simulink model "SimulationDroneSetup"  (R2025a)
settings: Solver=ode15s  StartTime=0.0  StopTime=3  FixedStep=0.03  RelTol=1e-3
InitFcn:
  | %% System Constants
  | 
  | % mass
  | m = 0.12635;
  | 
  | % graviational constant
  | g = 9.81;
  | 
  | % Moment of inertia
  | I_XX = 0.00016159;
  | I_YY = 0.00016466;
  | I_ZZ = 0.00026144;
  | 
  | % thrust and power factor - needs to be measured
  | c_t = 2.07732E-05;
  | c_p = 2.76277E-06;
  | 
  | % https://en.wikipedia.org/wiki/Density_of_air
  | rho = 1.225;
  | 
  | % surface area of a propeller - estimation based on half of circle area
  | diameter = 0.04;
  | A = pi * (diameter/2)^2 / 2;
  | 
  | % chord length - needs to be measured
  | r = 0.008;
  | 
  | %Thrust coefficient
  | b = c_t * rho * A * r^2;
  | 
  | %Torque drag coefficient
  | d_t = c_p * rho * A * r^3;
  | 
  | %Distance from CoG to propeller axis
  | l = 0.104707;
  | 
  | J_TP = 0.0041979;
settings Model: PacingRate=100  Creator=tobia  LastModifiedBy=dma

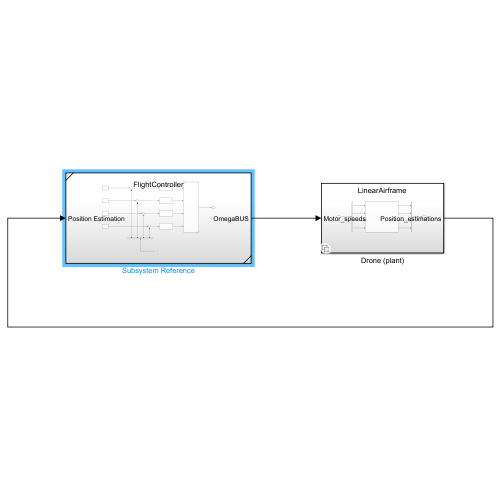
[thumbnail: Simulink's stored preview of the top-level diagram]
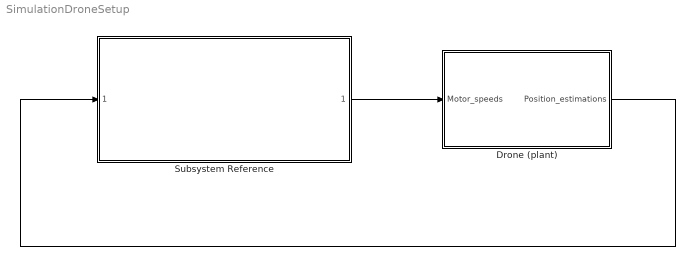
== system SimulationDroneSetup ==
  Drone (plant) : Subsystem  Variant=on
  Subsystem Reference : Subsystem  ReferencedSubsystem=FlightController
  wires:
  Subsystem Reference/1 -> Drone (plant)/1(Motor_speeds)
  Drone (plant)/1(Position_estimations) -> Subsystem Reference/1

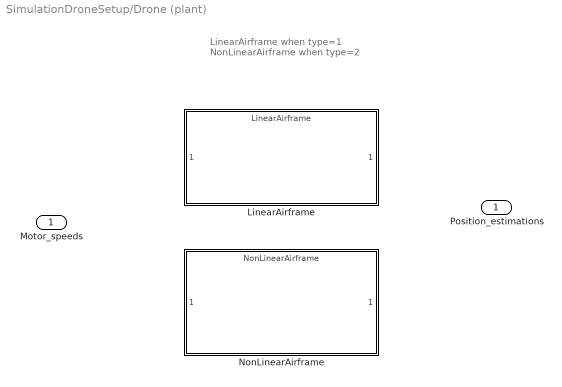
== system SimulationDroneSetup/Drone (plant) ==
  note: LinearAirframe when type=1
      | NonLinearAirframe when type=2
  Motor_speeds : Inport
  LinearAirframe : ModelReference  ModelNameDialog=LinearAirframe.slx  SimulationMode=Normal  VariantControl=type==1  ModelReferenceVersion=1.16
  NonLinearAirframe : ModelReference  ModelNameDialog=NonLinearAirframe.slx  SimulationMode=Normal  VariantControl=type==2  ModelReferenceVersion=1.5
  Position_estimations : Outport
